simulink model "XYZ_selector"  (R2024b)
settings: Solver=VariableStepAuto  StartTime=0.0  StopTime=10.0  RelTol=1e-3
settings Model: Creator=罗芳成  LastModifiedBy=罗芳成

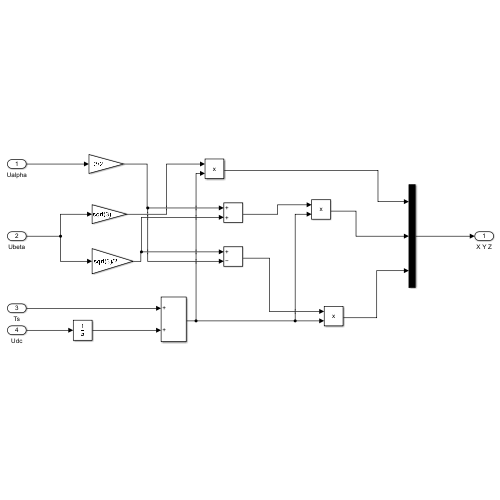
[thumbnail: Simulink's stored preview of the top-level diagram]
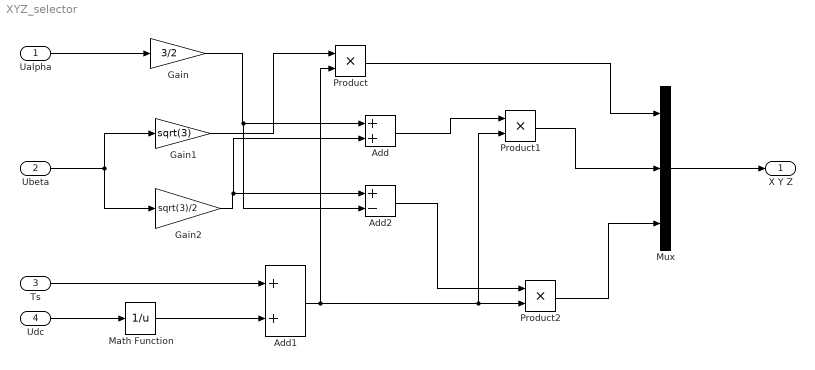
== system XYZ_selector ==
  Ualpha : Inport
  Ubeta : Inport  Port=2
  Ts : Inport  Port=3
  Udc : Inport  Port=4
  Add : Sum
  Add1 : Sum
  Add2 : Sum  Inputs=+-
  Gain : Gain  Gain=3/2
  Gain1 : Gain  Gain=sqrt(3)
  Gain2 : Gain  Gain=sqrt(3)/2
  Math Function : Math  Operator=reciprocal
  Mux : Mux  Inputs=3
  Product : Product
  Product1 : Product
  Product2 : Product
  X Y Z : Outport
  wires:
  Ualpha/1 -> Gain/1
  Ubeta/1 -> Gain1/1, Gain2/1
  Udc/1 -> Math Function/1
  Math Function/1 -> Add1/2
  Ts/1 -> Add1/1
  Gain1/1 -> Product/1
  Add1/1 -> Product2/2, Product1/2, Product/2
  Gain/1 -> Add2/2, Add/1
  Product/1 -> Mux/1
  Gain2/1 -> Add/2, Add2/1
  Add/1 -> Product1/1
  Add2/1 -> Product2/1
  Product1/1 -> Mux/2
  Product2/1 -> Mux/3
  Mux/1 -> X Y Z/1
